simulink model "mulplexuser"  (R2020a)
settings: Solver=VariableStepAuto  StartTime=0.0  StopTime=10.0  RelTol=1e-3
libraries: commrandsrc3 x6, commseqgen3 x6, dsparch4 x3, commsink2 x3, commutil2 x2, commdigbbndpm3 x2, commchan3 x1
settings Model: Creator=xxy15334437753  LastModifiedBy=xxy15334437753

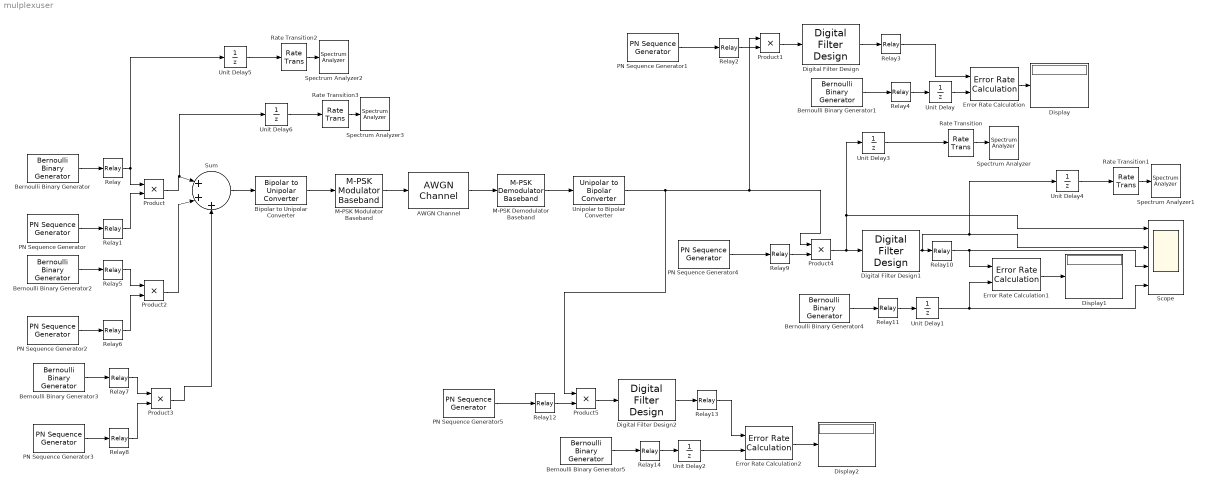
== system mulplexuser ==
  AWGN Channel : commchan3/AWGN Channel  InputProcessing=Columns as channels (frame based)  seed=67  noiseMode="Signal to noise ratio  (SNR)"  EbNodB=10  EsNodB=10  SNRdB=10  bitsPerSym=1  Ps=1  Tsym=1  variance=1
  Bernoulli Binary Generator : commrandsrc3/Bernoulli Binary Generator  ProbabilityOfZero=0.5  SeedSource=Parameter  Seed=67  SampleTime=6e-4  SamplesPerFrame=1  OutputDataType=double  SimulateUsing=Interpreted execution
  Bernoulli Binary Generator1 : commrandsrc3/Bernoulli Binary Generator  ProbabilityOfZero=0.5  SeedSource=Parameter  Seed=67  SampleTime=6e-4  SamplesPerFrame=1  OutputDataType=double  SimulateUsing=Interpreted execution
  Bernoulli Binary Generator2 : commrandsrc3/Bernoulli Binary Generator  ProbabilityOfZero=0.5  SeedSource=Parameter  Seed=77  SampleTime=6e-4  SamplesPerFrame=1  OutputDataType=double  SimulateUsing=Interpreted execution
  Bernoulli Binary Generator3 : commrandsrc3/Bernoulli Binary Generator  ProbabilityOfZero=0.5  SeedSource=Parameter  Seed=87  SampleTime=6e-4  SamplesPerFrame=1  OutputDataType=double  SimulateUsing=Interpreted execution
  Bernoulli Binary Generator4 : commrandsrc3/Bernoulli Binary Generator  ProbabilityOfZero=0.5  SeedSource=Parameter  Seed=77  SampleTime=6e-4  SamplesPerFrame=1  OutputDataType=double  SimulateUsing=Interpreted execution
  Bernoulli Binary Generator5 : commrandsrc3/Bernoulli Binary Generator  ProbabilityOfZero=0.5  SeedSource=Parameter  Seed=87  SampleTime=6e-4  SamplesPerFrame=1  OutputDataType=double  SimulateUsing=Interpreted execution
  Bipolar to Unipolar Converter : commutil2/Bipolar to Unipolar Converter  M=8  polarity=Positive  dataType=Inherit via internal rule
      settings: SourceProductBaseCode=CM
  Digital Filter Design : dsparch4/Digital Filter Design  mwdsp_browser_bugfix_var=off
  Digital Filter Design1 : dsparch4/Digital Filter Design  mwdsp_browser_bugfix_var=off
  Digital Filter Design2 : dsparch4/Digital Filter Design  mwdsp_browser_bugfix_var=off
  Display : Display
  Display1 : Display
  Display2 : Display
  Error Rate Calculation : commsink2/Error Rate Calculation  N=0  st_delay=0  cp_mode=Entire frame  subframe=[]  PMode=Port  WsName=ErrorVec  RsMode2=off  stop=off  numErr=100  maxBits=1e6
  Error Rate Calculation1 : commsink2/Error Rate Calculation  N=0  st_delay=0  cp_mode=Entire frame  subframe=[]  PMode=Port  WsName=ErrorVec  RsMode2=off  stop=off  numErr=100  maxBits=1e6
  Error Rate Calculation2 : commsink2/Error Rate Calculation  N=0  st_delay=0  cp_mode=Entire frame  subframe=[]  PMode=Port  WsName=ErrorVec  RsMode2=off  stop=off  numErr=100  maxBits=1e6
  M-PSK Demodulator Baseband : commdigbbndpm3/M-PSK Demodulator Baseband  M=8  OutType=Integer  DecType=Hard decision  VarSource=Dialog  Variance=1  Dec=Gray  Mapping=[0:7]  Ph=pi/8  outDtype1=Inherit via internal rule  outDtype2=Inherit via internal rule  derotateFactorWordLen=16  derotateFactorDataTypeStr=Inherit: Same word length as input  derotateFactorLastDataTypeStr=Inherit: Same word length as input
  M-PSK Modulator Baseband : commdigbbndpm3/M-PSK Modulator Baseband  M=8  InType=Integer  Enc=Gray  Mapping=[0:7]  Ph=pi/8  outDtype=double  outWordLen=16  outUDDataType=sfix(16)  outFracLenMode=Best precision  outFracLen=15  outDataTypeStr=double  outLastDataTypeStr=double
  PN Sequence Generator : commseqgen3/PN Sequence Generator  poly='z^6 + z + 1'  ini_sta=[0 0 0 0 0 1]  outBitMaskSource=Dialog parameter  shift=0  outVarSiz=off  maxOutSizeMode=Dialog parameter  maxOutSize=[10 1]  Ts=1/50000  sampPerFrame=1  reset=off  bitPackedOutputs=off  outDataType=double  numPackedBits=8  bitPackDataSigned=off  bitPackedOutDType=double
  PN Sequence Generator1 : commseqgen3/PN Sequence Generator  poly='z^6 + z + 1'  ini_sta=[0 0 0 0 0 1]  outBitMaskSource=Dialog parameter  shift=0  outVarSiz=off  maxOutSizeMode=Dialog parameter  maxOutSize=[10 1]  Ts=2e-5  sampPerFrame=1  reset=off  bitPackedOutputs=off  outDataType=double  numPackedBits=8  bitPackDataSigned=off  bitPackedOutDType=double
  PN Sequence Generator2 : commseqgen3/PN Sequence Generator  poly='z^6 + z + 1'  ini_sta=[0 0 0 0 1 1]  outBitMaskSource=Dialog parameter  shift=0  outVarSiz=off  maxOutSizeMode=Dialog parameter  maxOutSize=[10 1]  Ts=2e-5  sampPerFrame=1  reset=off  bitPackedOutputs=off  outDataType=double  numPackedBits=8  bitPackDataSigned=off  bitPackedOutDType=double
  PN Sequence Generator3 : commseqgen3/PN Sequence Generator  poly='z^6 + z + 1'  ini_sta=[0 0 0 1 1 1]  outBitMaskSource=Dialog parameter  shift=0  outVarSiz=off  maxOutSizeMode=Dialog parameter  maxOutSize=[10 1]  Ts=2e-5  sampPerFrame=1  reset=off  bitPackedOutputs=off  outDataType=double  numPackedBits=8  bitPackDataSigned=off  bitPackedOutDType=double
  PN Sequence Generator4 : commseqgen3/PN Sequence Generator  poly='z^6 + z + 1'  ini_sta=[0 0 0 0 1 1]  outBitMaskSource=Dialog parameter  shift=0  outVarSiz=off  maxOutSizeMode=Dialog parameter  maxOutSize=[10 1]  Ts=2e-5  sampPerFrame=1  reset=off  bitPackedOutputs=off  outDataType=double  numPackedBits=8  bitPackDataSigned=off  bitPackedOutDType=double
  PN Sequence Generator5 : commseqgen3/PN Sequence Generator  poly='z^6 + z + 1'  ini_sta=[0 0 0 1 1 1]  outBitMaskSource=Dialog parameter  shift=0  outVarSiz=off  maxOutSizeMode=Dialog parameter  maxOutSize=[10 1]  Ts=2e-5  sampPerFrame=1  reset=off  bitPackedOutputs=off  outDataType=double  numPackedBits=8  bitPackDataSigned=off  bitPackedOutDType=double
  Product{,1..5} (6 alike) : Product
  Rate Transition : RateTransition  OutPortSampleTime=1/200000
  Rate Transition1 : RateTransition  OutPortSampleTime=8e-5
  Rate Transition2 : RateTransition  OutPortSampleTime=3e-5
  Rate Transition3 : RateTransition  OutPortSampleTime=1/200000
  Relay{,1..2,4..9,11..12,14} (12 alike) : Relay  OnSwitchValue=0.9  OffSwitchValue=0.1  OffOutputValue=-1
  Relay10 : Relay  OnSwitchValue=0  OffSwitchValue=0  OffOutputValue=-1
  Relay13 : Relay  OnSwitchValue=0  OffSwitchValue=0  OffOutputValue=-1
  Relay3 : Relay  OnSwitchValue=0  OffSwitchValue=0  OffOutputValue=-1
  Scope : Scope  NumInputPorts=4
  Spectrum Analyzer{,1..3} (4 alike) : SpectrumAnalyzer
  Sum : Sum  Inputs=|+++
  Unipolar to Bipolar Converter : commutil2/Unipolar to Bipolar Converter  M=8  polarity=Positive  dataType=Inherit via internal rule
  Unit Delay{,1..6} (7 alike) : UnitDelay  SampleTime=-1  HasFrameUpgradeWarning=on
  wires:
  Bernoulli Binary Generator/1 -> Relay/1
  PN Sequence Generator/1 -> Relay1/1
  Relay1/1 -> Product/2
  M-PSK Modulator Baseband/1 -> AWGN Channel/1
  Sum/1 -> Bipolar to Unipolar Converter/1
  Bipolar to Unipolar Converter/1 -> M-PSK Modulator Baseband/1
  M-PSK Demodulator Baseband/1 -> Unipolar to Bipolar Converter/1
  AWGN Channel/1 -> M-PSK Demodulator Baseband/1
  PN Sequence Generator1/1 -> Relay2/1
  Relay2/1 -> Product1/2
  Product1/1 -> Digital Filter Design/1
  Digital Filter Design/1 -> Relay3/1
  Bernoulli Binary Generator1/1 -> Relay4/1
  Relay4/1 -> Unit Delay/1
  Unit Delay/1 -> Error Rate Calculation/2
  Relay3/1 -> Error Rate Calculation/1
  Error Rate Calculation/1 -> Display/1
  Relay6/1 -> Product2/2
  Product2/1 -> Sum/2
  PN Sequence Generator2/1 -> Relay6/1
  Relay5/1 -> Product2/1
  Bernoulli Binary Generator2/1 -> Relay5/1
  Relay8/1 -> Product3/2
  Product3/1 -> Sum/3
  PN Sequence Generator3/1 -> Relay8/1
  Relay7/1 -> Product3/1
  Bernoulli Binary Generator3/1 -> Relay7/1
  Relay11/1 -> Unit Delay1/1
  Error Rate Calculation1/1 -> Display1/1
  Relay9/1 -> Product4/2
  Digital Filter Design1/1 -> Unit Delay4/1, Scope/2, Relay10/1
  PN Sequence Generator4/1 -> Relay9/1
  Relay10/1 -> Scope/3, Error Rate Calculation1/1
  Product4/1 -> Unit Delay3/1, Scope/1, Digital Filter Design1/1
  Unit Delay1/1 -> Scope/4, Error Rate Calculation1/2
  Bernoulli Binary Generator4/1 -> Relay11/1
  Relay14/1 -> Unit Delay2/1
  Error Rate Calculation2/1 -> Display2/1
  Relay12/1 -> Product5/2
  Digital Filter Design2/1 -> Relay13/1
  PN Sequence Generator5/1 -> Relay12/1
  Relay13/1 -> Error Rate Calculation2/1
  Unipolar to Bipolar Converter/1 -> Product5/1, Product4/1, Product1/1
  Product5/1 -> Digital Filter Design2/1
  Unit Delay2/1 -> Error Rate Calculation2/2
  Bernoulli Binary Generator5/1 -> Relay14/1
  Rate Transition/1 -> Spectrum Analyzer/1
  Rate Transition1/1 -> Spectrum Analyzer1/1
  Unit Delay4/1 -> Rate Transition1/1
  Unit Delay3/1 -> Rate Transition/1
  Unit Delay5/1 -> Rate Transition2/1
  Relay/1 -> Unit Delay5/1, Product/1
  Rate Transition2/1 -> Spectrum Analyzer2/1
  Unit Delay6/1 -> Rate Transition3/1
  Product/1 -> Unit Delay6/1, Sum/1
  Rate Transition3/1 -> Spectrum Analyzer3/1
